simulink model "SCex2simulink"  (R2024b)
settings: Solver=VariableStepAuto  StartTime=0.0  StopTime=100  RelTol=1e-3
values from neighbouring files (symbols this model uses):
  A = [  0       1       0       0 ... (first row only)    [SCex2.m]    (also in SCex3_3.m = [0, 1; -(k/m), -(b/m)])
  B = [ 0; k1/m1; 0; 0 ]    [SCex2.m]    (also in SCex3_3.m = [2.4; -1.6])
  C = [ 1 0 0 0; 0 0 1 0 ]    [SCex2.m]    (also in SCex3_3.m = [1, 0 ; 0, 1])
  D = [ 0; 0 ]    [SCex2.m]    (also in SCex3_3.m = [0; 0])
settings Model: Creator=pedro  LastModifiedBy=pedro

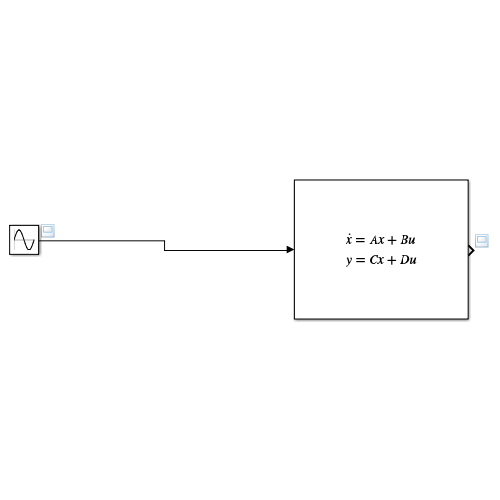
[thumbnail: Simulink's stored preview of the top-level diagram]
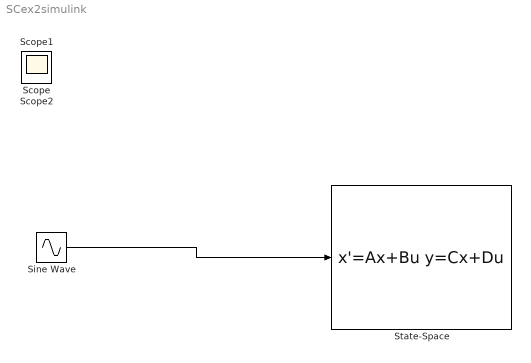
== system SCex2simulink ==
  Sine Wave : Sin  SampleTime=0
  State-Space : StateSpace  A=A  B=B  C=C  D=D  InitialCondition=0
  Scope : Scope
  Scope1 : Scope
  Scope2 : Scope
  wires:
  Sine Wave/1 -> State-Space/1
